simulink model "Closed_Loop_System_With_P_Controller"  (R2023a)
settings: Solver=FixedStepDiscrete  StartTime=0.0  StopTime=10  FixedStep=0.001  RelTol=1e-3  EnableMultiTasking=on
libraries: arduinolib x4
settings Model: ExtModeTrigDuration=2  Creator=Mohamed Ezzelrgal  LastModifiedBy=Mohamed Ezzelrgal
settings OptimizationCC: EnhancedBackFolding=on  PassReuseOutputArgsAs=Individual arguments  ZeroExternalMemoryAtStartup=off  ZeroInternalMemoryAtStartup=off  MaxStackSize=64  OptimizeBlockOrder=speed  DifferentSizesBufferReuse=on  OptimizationCustomize=off  EfficientTunableParamExpr=on
settings DebuggingCC: ParameterTunabilityLossMsg=error
settings HardwareCC: ProdBitPerInt=16  ProdBitPerPointer=16  ProdBitPerSizeT=16  ProdBitPerPtrDiffT=16  ProdLargestAtomicFloat=None  ProdWordSize=8  ProdHWDeviceType=Atmel->AVR
settings SFSimCC: MATLABDynamicMemAlloc=off
settings RTWCC: Description=Embedded Coder  SystemTargetFile=ert.tlc  HardwareBoard=Arduino Uno  TemplateMakefile=ert_default_tmf  Toolchain=Arduino AVR  BuildConfiguration=Faster Runs
settings CodeAppCC: ForceParamTrailComments=on  IgnoreCustomStorageClasses=off  OperatorAnnotations=on  SimulinkDataObjDesc=on  SFDataObjDesc=on  InsertBlockDesc=on
settings ERTTargetCC: SupportContinuousTime=on  SupportVariableSizeSignals=on  ExtModeTransport=3  ExtModeStaticAlloc=on  ExtModeAutomaticAllocSize=off  ExtModeStaticAllocSize=250  ExtModeMexFile=ext_xcp  ExtModeIntrfLevel=Level2 - Open

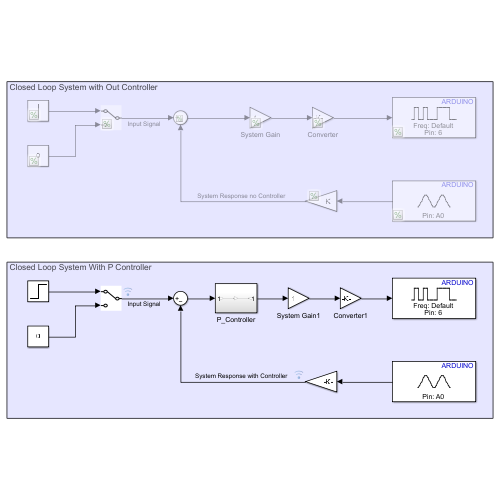
[thumbnail: Simulink's stored preview of the top-level diagram]
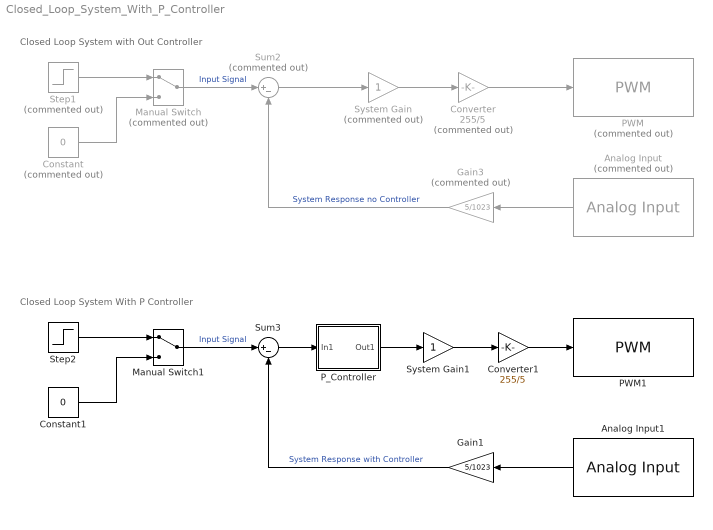
== system Closed_Loop_System_With_P_Controller ==
  note: Closed Loop System With P Controller
  note: Closed Loop System with Out Controller
  Analog Input : arduinolib/Analog Input  Commented=on  pinNumber=0  ReadResultsOnly=off  ConversionTriggerSource=Software  ExternalTriggerType=uint32( 0 )  OutputDataType=uint16  EnableConversionCompleteNotify=off  EnableOuputStatus=off  SampleTime=-1  blockPlatform=arduino
  Analog Input1 : arduinolib/Analog Input  pinNumber=0  ReadResultsOnly=off  ConversionTriggerSource=Software  ExternalTriggerType=uint32( 0 )  OutputDataType=uint16  EnableConversionCompleteNotify=off  EnableOuputStatus=off  SampleTime=-1  blockPlatform=arduino
  Constant : Constant  Commented=on  Value=0
  Constant1 : Constant  Value=0
  Converter : Gain  Commented=on  Gain=255/5
  Converter1 : Gain  Gain=255/5
  Gain1 : Gain  Gain=5/1023
  Gain3 : Gain  Commented=on  Gain=5/1023
  Manual Switch : ManualSwitch  Commented=on
  Manual Switch1 : ManualSwitch
  PWM : arduinolib/PWM  Commented=on  pinNumber=6  frequencyType=Default  desiredFrequency=490.2  achievableFrequency=490.2
  PWM1 : arduinolib/PWM  pinNumber=6  frequencyType=Default  desiredFrequency=490.2  achievableFrequency=490.2
  P_Controller : Subsystem
  Step1 : Step  Commented=on  SampleTime=0
  Step2 : Step  SampleTime=0
  Sum2 : Sum  Commented=on  Inputs=|+-
  Sum3 : Sum  Inputs=|+-
  System Gain : Gain  Commented=on
  System Gain1 : Gain
  wires:
  Converter/1 -> PWM/1
  System Gain/1 -> Converter/1
  Step1/1 -> Manual Switch/1
  Constant/1 -> Manual Switch/2
  Analog Input/1 -> Gain3/1
  Gain3/1 -> Sum2/2  "System Response no Controller"
  Sum2/1 -> System Gain/1
  Manual Switch/1 -> Sum2/1  "Input Signal"
  Manual Switch1/1 -> Sum3/1  "Input Signal"
  Sum3/1 -> P_Controller/1(In1)
  Gain1/1 -> Sum3/2  "System Response with Controller"
  Analog Input1/1 -> Gain1/1
  Constant1/1 -> Manual Switch1/2
  Step2/1 -> Manual Switch1/1
  System Gain1/1 -> Converter1/1
  Converter1/1 -> PWM1/1
  P_Controller/1(Out1) -> System Gain1/1

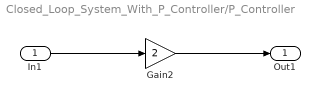
== system Closed_Loop_System_With_P_Controller/P_Controller ==
  In1 : Inport
  Gain2 : Gain  Gain=2
  Out1 : Outport
  wires:
  In1/1 -> Gain2/1
  Gain2/1 -> Out1/1
